simulink model "On_Board_Computer"  (R2024a)
settings: Solver=FixedStepAuto  StartTime=0.0  StopTime=10  FixedStep=sampleTime  RelTol=1e-3
values from neighbouring files (symbols this model uses):
  gains = gainBuilder(kP, kI, kD)    [Data.m]
  params = struct()    [Data.m]
  Q = 0.*eye(12).*1e-0    [Data.m]
  R = diag([(sigma_acc^2).*ones(3,1);      (sigma_gyro^2).*ones(3,1)])    [Data.m]
  sampleTime = 0.01    [Data.m]
libraries: sharedTrackingLibrary x1
settings Model: Creator=matteocolussi  LastModifiedBy=matteocolussi
settings DataIOCC: SaveOutput=off  SaveTime=off
settings DebuggingCC: ParameterPrecisionLossMsg=none
settings ModelReferenceCC: UseModelRefSolver=on

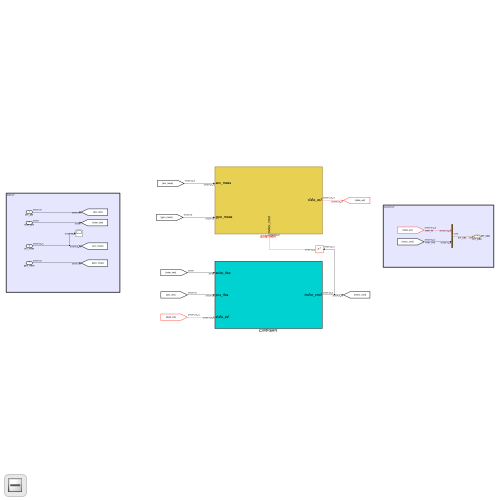
[thumbnail: Simulink's stored preview of the top-level diagram]
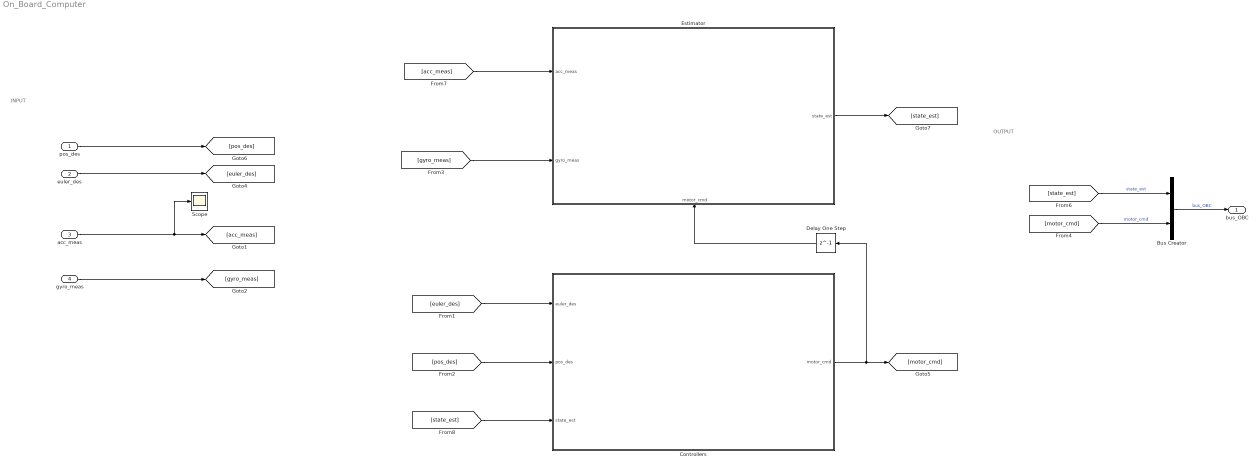
== system On_Board_Computer ==
  note: INPUT
  note: OUTPUT
  pos_des : Inport  OutDataTypeStr=double  PortDimensions=3
  euler_des : Inport  Port=2  OutDataTypeStr=double  PortDimensions=1
  acc_meas : Inport  Port=3  OutDataTypeStr=double  PortDimensions=[3 1]  SampleTime=0
  gyro_meas : Inport  Port=4  OutDataTypeStr=double  PortDimensions=3  SampleTime=0
  Bus Creator : BusCreator  Inputs=2  OutDataTypeStr=Bus: bus_OBC
  Controllers : Subsystem
  Delay One Step : Delay  DelayLength=1
  Estimator : Subsystem
      settings: PortSchema="{\"entries\":[{\"content\":{\"sides\":[{\"content\":{\"connectorIds\":[\"In1\",\"In2\"]},\"type\":\"ConnectorPlacement.EquallySpacedRectSide\",\"uuid\":\"d977f4b7-c562-4aca-a182-8854d6f84319\"},{\"content\":{\"connectorIds\":[\"Out1\"],\"side\":\"RIGHT\"},\"type\":\"ConnectorPlacement.EquallySpacedRectSide\",\"uuid\":\"5ec2f9b4-7086-4916-9bca-a6bf4e760209\"},{\"content\":{\"side\":\"TOP\"},\"type\":\"ConnectorPlacement.EquallySpacedRectSide\",\"uuid\":\"f97c9147-b60d-497a-8876-5f5880fb5fe3\"},{\"content\":{\"connectorIds\":[\"In3\"],\"side\":\"BOTTOM\"},\"type\":\"ConnectorPlacement.EquallySpacedRectSide\",\"uuid\":\"4e01cfcf-7d04-45a0-a360-97a990265c59\"}]},\"type\":\"ConnectorPlacement.EquallySpacedConnector\",\"uuid\":\"f1c31a70-7567-4742-915b-d219842d21d0\"}],\"packageUris\":[\"http://schema.mathworks.com/mf0/Connector/R2020b\"],\"version\":\"1.0\"}"
  Scope : Scope
  bus_OBC : Outport  SignalName=bus_OBC  OutDataTypeStr=Bus: bus_OBC
  wires:
  [euler_des] -> Controllers/1(euler_des)
  [gyro_meas] -> Estimator/2(gyro_meas)
  [acc_meas] -> Estimator/1(acc_meas)
  [pos_des] -> Controllers/2(pos_des)
  Estimator/1(state_est) -> [state_est]
  Controllers/1(motor_cmd) -> Delay One Step/1, [motor_cmd]
  Delay One Step/1 -> Estimator/3(motor_cmd)
  [state_est] -> Controllers/3(state_est)
  [state_est] -> Bus Creator/1  "state_est"
  [motor_cmd] -> Bus Creator/2  "motor_cmd"
  Bus Creator/1 -> bus_OBC/1  "bus_OBC"
  pos_des/1 -> [pos_des]
  euler_des/1 -> [euler_des]
  acc_meas/1 -> [acc_meas], Scope/1
  gyro_meas/1 -> [gyro_meas]

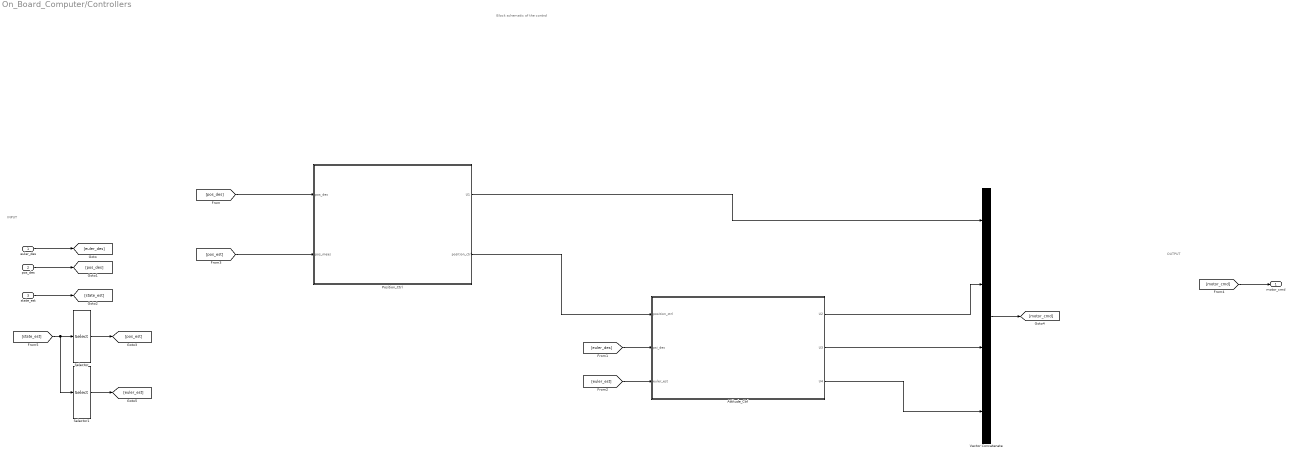
== system On_Board_Computer/Controllers ==
  note: INPUT
  note: OUTPUT
  note: Block schematic of the control
  euler_des : Inport
  pos_des : Inport  Port=2
  state_est : Inport  Port=3
  Attitude_Ctrl : Subsystem
  Position_Ctrl : Subsystem
  Selector : Selector  InputPortWidth=12  IndexOptions=Index vector (dialog)  Indices=1:3  OutputSizes=1
  Selector1 : Selector  InputPortWidth=12  IndexOptions=Index vector (dialog)  Indices=7:9  OutputSizes=1
  Vector Concatenate : Concatenate  NumInputs=4
  motor_cmd : Outport
  wires:
  [euler_des] -> Attitude_Ctrl/2(psi_des)
  Vector Concatenate/1 -> [motor_cmd]
  Attitude_Ctrl/3(U4) -> Vector Concatenate/4
  Attitude_Ctrl/2(U3) -> Vector Concatenate/3
  Attitude_Ctrl/1(U2) -> Vector Concatenate/2
  Position_Ctrl/1(U1) -> Vector Concatenate/1
  Position_Ctrl/2(position_ctrl) -> Attitude_Ctrl/1(position_ctrl)
  [pos_des] -> Position_Ctrl/1(pos_des)
  [pos_est] -> Position_Ctrl/2(pos_meas)
  [motor_cmd] -> motor_cmd/1
  [euler_est] -> Attitude_Ctrl/3(euler_est)
  state_est/1 -> [state_est]
  Selector/1 -> [pos_est]
  pos_des/1 -> [pos_des]
  euler_des/1 -> [euler_des]
  [state_est] -> Selector1/1, Selector/1
  Selector1/1 -> [euler_est]

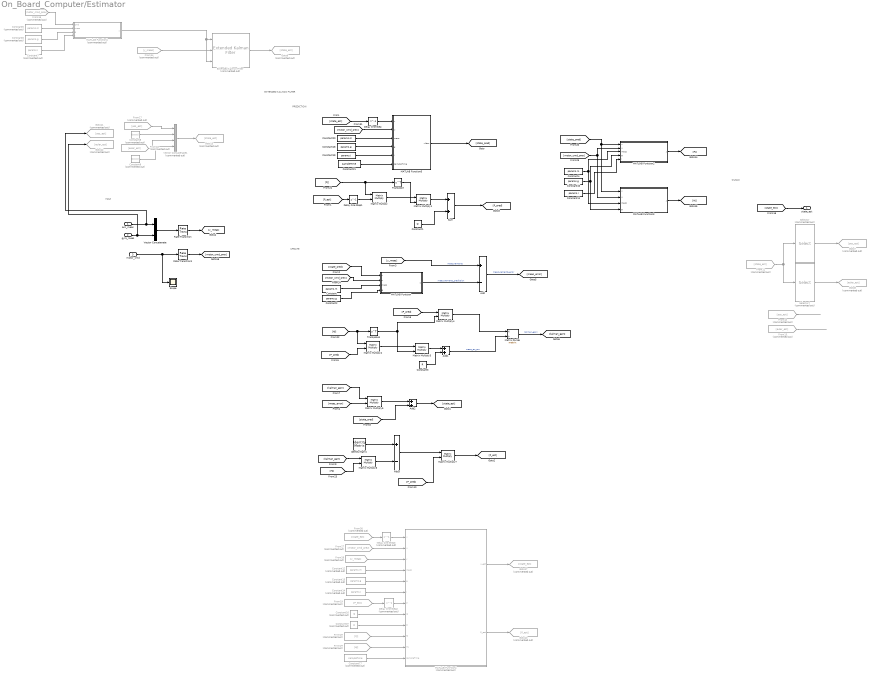
== system On_Board_Computer/Estimator ==
  note: Output
  note: Input
  note: UPDATE
  note: PREDICTION
  note: EXTENDED KALMAN FILTER
  acc_meas : Inport
  gyro_meas : Inport  Port=2
  motor_cmd : Inport  Port=3
  Add : Sum  Inputs=+-
  Add1 : Sum
  Add2 : Sum
  Add3 : Sum  Inputs=+-
  Constant : Constant  Value=params.m
  Constant1 : Constant  Value=Q
  Constant10 : Constant  Value=params.g
  Constant11 : Constant  Value=params.I
  Constant12 : Constant  Commented=on  Value=params.m
  Constant13 : Constant  Commented=on  Value=params.g
  Constant14 : Constant  Commented=on  Value=params.I
  Constant15 : Constant  Commented=on  Value=R
  Constant16 : Constant  Commented=on  Value=Q
  Constant17 : Constant  Commented=on  Value=sampleTime
  Constant18 : Constant  Value=params.g
  Constant19 : Constant  Value=params.I
  Constant2 : Constant  Value=params.g
  Constant20 : Constant  Value=params.m
  Constant21 : Constant  Value=sampleTime
  Constant3 : Constant  Value=R
  Constant4 : Constant  Value=params.m
  Constant5 : Constant  Commented=on  Value=params.m
  Constant6 : Constant  Commented=on  Value=params.g
  Constant7 : Constant  Commented=on  Value=params.I
  Constant8 : Constant  Commented=on  Value=[0;0;0]
  Constant9 : Constant  Commented=on  Value=[0;0;0]
  Delay One Step : Delay  DelayLength=1
  Delay One Step1 : Delay  DelayLength=1
  Delay One Step2 : Delay  Commented=on  DelayLength=1
  Delay One Step3 : Delay  Commented=on  DelayLength=1
  Extended Kalman Filter : sharedTrackingLibrary/Extended Kalman Filter  Commented=on  StateTransitionFcn=stateFunction  HasStateTransitionJacobianFcn=off  HasAdditiveProcessNoise=Additive  ProcessNoise=Q  HasTimeVaryingProcessNoise=off  HasStateTransitionFcnExtraArgument=1  InitialState=zeros(12,1)  InitialStateCovariance=P_est  MeasurementFcn1=measFunction  HasMeasurementJacobianFcn1=off  HasMeasurementEnablePort1=off  HasAdditiveMeasurementNoise1=Additive  MeasurementNoise1=R  HasTimeVaryingMeasurementNoise1=off  HasMeasurementFcnExtraArgument1=1  HasMeasurementWrapping1=off  MeasurementFcn2=myMeasurementFcn  HasMeasurementJacobianFcn2=off  HasMeasurementEnablePort2=off  HasAdditiveMeasurementNoise2=Additive  MeasurementNoise2=1  HasTimeVaryingMeasurementNoise2=off  HasMeasurementFcnExtraArgument2=0  HasMeasurementWrapping2=off  MeasurementFcn3=myMeasurementFcn  HasMeasurementJacobianFcn3=off  HasMeasurementEnablePort3=off  HasAdditiveMeasurementNoise3=Additive  MeasurementNoise3=1  HasTimeVaryingMeasurementNoise3=off  HasMeasurementFcnExtraArgument3=0  HasMeasurementWrapping3=off  MeasurementFcn4=myMeasurementFcn  HasMeasurementJacobianFcn4=off  HasMeasurementEnablePort4=off  HasAdditiveMeasurementNoise4=Additive  MeasurementNoise4=1  HasTimeVaryingMeasurementNoise4=off  HasMeasurementFcnExtraArgument4=0  HasMeasurementWrapping4=off  MeasurementFcn5=myMeasurementFcn  HasMeasurementJacobianFcn5=off  HasMeasurementEnablePort5=off  HasAdditiveMeasurementNoise5=Additive  MeasurementNoise5=1  HasTimeVaryingMeasurementNoise5=off  HasMeasurementFcnExtraArgument5=0  HasMeasurementWrapping5=off  EnableMultirate=off  StateTransitionFcnSampleTime=1  MeasurementFcn1SampleTime=1  MeasurementFcn2SampleTime=1  MeasurementFcn3SampleTime=1  MeasurementFcn4SampleTime=1  MeasurementFcn5SampleTime=1  UseCurrentEstimator=on  OutputStateCovariance=off  DataType=double  SampleTime=sampleTime  NumberOfMeasurements=1
  From11 : From  Commented=on  GotoTag=state_est
  From12 : From  Commented=on  GotoTag=pos_est
  From13 : From  Commented=on  GotoTag=euler_est
  From14 : From  Commented=on  GotoTag=y_meas
  From15 : From  Commented=on  GotoTag=motor_cmd_prev
  From17 : From  Commented=on  GotoTag=pos_est
  From18 : From  Commented=on  GotoTag=euler_est
  From19 : From  Commented=on  GotoTag=P_est
  From26 : From  Commented=on  GotoTag=y_meas
  From27 : From  Commented=on  GotoTag=motor_cmd_prev
  From28 : From  Commented=on  GotoTag=FJ
  From29 : From  Commented=on  GotoTag=HJ
  From30 : From  Commented=on  GotoTag=state_est
  Goto10 : Goto  Commented=on  GotoTag=P_est
  Goto11 : Goto  Commented=on  GotoTag=pos_est
  Goto12 : Goto  Commented=on  GotoTag=euler_est
  Goto13 : Goto  Commented=on  GotoTag=state_est
  Goto17 : Goto  Commented=on  GotoTag=state_est
  Goto7 : Goto  Commented=on  GotoTag=pos_est
  Goto8 : Goto  Commented=on  GotoTag=euler_est
  Goto9 : Goto  Commented=on  GotoTag=state_est
  IdentityMatrix : IdentityMatrix  OutputDimensions=[12,12]  SampleTime=inf
  MATLAB Function : MATLAB Function  TreatAsAtomicUnit=on
  MATLAB Function1 : MATLAB Function  Commented=on  TreatAsAtomicUnit=on
  MATLAB Function2 : MATLAB Function  TreatAsAtomicUnit=on
  MATLAB Function3 : MATLAB Function  TreatAsAtomicUnit=on
  MATLAB Function4 : MATLAB Function  Commented=on  TreatAsAtomicUnit=on
  MATLAB Function5 : MATLAB Function  TreatAsAtomicUnit=on
  Matrix Divide : Product  Inputs=*/  Multiplication=Matrix(*)
  Matrix Multiply{,1..7} (8 alike) : Product  Multiplication=Matrix(*)
  Rate Transition : RateTransition  OutPortSampleTime=sampleTime
  Rate Transition1 : RateTransition  OutPortSampleTime=sampleTime
  Scope : Scope
  Selector : Selector  Commented=on  InputPortWidth=12  IndexOptions=Index vector (dialog)  Indices=1:3  OutputSizes=1
  Selector1 : Selector  Commented=on  InputPortWidth=12  IndexOptions=Index vector (dialog)  Indices=7:9  OutputSizes=1
  Sum : Sum
  Transpose : Math  Operator=transpose
  Transpose1 : Math  Operator=transpose
  Vector Concatenate : Concatenate
  Vector Concatenate1 : Concatenate  Commented=on  NumInputs=4
  state_est : Outport
  wires:
  acc_meas/1 -> Vector Concatenate/1, Goto11/1
  gyro_meas/1 -> Vector Concatenate/2, Goto12/1
  [state_est] -> Delay One Step/1
  Delay One Step/1 -> MATLAB Function5/1(x)
  [P_est] -> Delay One Step1/1
  Delay One Step1/1 -> Matrix Multiply/2
  Matrix Multiply/1 -> Matrix Multiply1/1
  [FJ] -> Transpose/1, Matrix Multiply/1
  Transpose/1 -> Matrix Multiply1/2
  Matrix Multiply1/1 -> Sum/1
  Constant1/1 -> Sum/2
  Sum/1 -> [P_pred]
  [state_pred] -> MATLAB Function/1(x)
  MATLAB Function/1(z) -> Add/2  "measurements_prediction"
  Vector Concatenate/1 -> Rate Transition/1
  [y_meas] -> Add/1  "measurements"
  Add/1 -> [meas_error]  "measurements_error"
  [P_pred] -> Matrix Multiply2/2
  [HJ] -> Matrix Multiply2/1, Transpose1/1
  Matrix Multiply2/1 -> Matrix Multiply3/1
  Transpose1/1 -> Matrix Multiply4/2, Matrix Multiply3/2
  Matrix Multiply3/1 -> Add1/1
  Constant3/1 -> Add1/2
  Add1/1 -> Matrix Divide/2  "meas_err_cov"
  [P_pred] -> Matrix Multiply4/1
  Matrix Multiply4/1 -> Matrix Divide/1
  Matrix Divide/1 -> [kalman_gain]  "kalman_gain"
  [meas_error] -> Matrix Multiply5/2
  [kalman_gain] -> Matrix Multiply5/1
  Matrix Multiply5/1 -> Add2/1
  [state_pred] -> Add2/2
  Add2/1 -> [state_est]
  IdentityMatrix/1 -> Add3/1
  [kalman_gain] -> Matrix Multiply6/1
  [HJ] -> Matrix Multiply6/2
  Matrix Multiply6/1 -> Add3/2
  Add3/1 -> Matrix Multiply7/1
  Matrix Multiply7/1 -> [P_est]
  [P_pred] -> Matrix Multiply7/2
  From11/1 -> Selector1/1, Selector/1
  Selector/1 -> Goto7/1
  Selector1/1 -> Goto8/1
  From12/1 -> ?
  From13/1 -> ?
  Extended Kalman Filter/1 -> Goto9/1
  motor_cmd/1 -> Scope/1, Rate Transition1/1
  From14/1 -> Extended Kalman Filter/2
  Rate Transition/1 -> [y_meas]
  Rate Transition1/1 -> [motor_cmd_prev]
  From15/1 -> MATLAB Function1/1(cmd)
  Constant5/1 -> MATLAB Function1/2(mass)
  Constant6/1 -> MATLAB Function1/3(g)
  Constant7/1 -> MATLAB Function1/4(I)
  MATLAB Function1/1(y) -> Extended Kalman Filter/3, Extended Kalman Filter/1
  [state_est] -> state_est/1
  From17/1 -> Vector Concatenate1/1
  Constant8/1 -> Vector Concatenate1/2
  From18/1 -> Vector Concatenate1/3
  Constant9/1 -> Vector Concatenate1/4
  Vector Concatenate1/1 -> Goto13/1
  [motor_cmd_prev] -> MATLAB Function3/2(u), MATLAB Function2/2(u)
  [state_pred] -> MATLAB Function3/1(x), MATLAB Function2/1(x)
  MATLAB Function2/1(J) -> [FJ]
  MATLAB Function3/1(J) -> [HJ]
  [motor_cmd_prev] -> MATLAB Function/2(u)
  Constant/1 -> MATLAB Function/3(mass)
  Constant2/1 -> MATLAB Function/4(g)
  Constant4/1 -> MATLAB Function3/3(mass), MATLAB Function2/3(mass)
  Constant10/1 -> MATLAB Function3/4(g), MATLAB Function2/4(g)
  Constant11/1 -> MATLAB Function2/5(I)
  MATLAB Function4/2(P_est) -> Goto10/1
  MATLAB Function4/1(x_est) -> Goto17/1
  From19/1 -> Delay One Step2/1
  Delay One Step2/1 -> MATLAB Function4/7(P)
  Constant13/1 -> MATLAB Function4/5(g)
  Constant12/1 -> MATLAB Function4/4(mass)
  Constant14/1 -> MATLAB Function4/6(I)
  From26/1 -> MATLAB Function4/3(y)
  From27/1 -> MATLAB Function4/2(u)
  Constant15/1 -> MATLAB Function4/9(R)
  Constant16/1 -> MATLAB Function4/8(Q)
  From28/1 -> MATLAB Function4/10(FJ)
  From29/1 -> MATLAB Function4/11(HJ)
  From30/1 -> Delay One Step3/1
  Delay One Step3/1 -> MATLAB Function4/1(x)
  Constant17/1 -> MATLAB Function4/12(sampleTime)
  MATLAB Function5/1(xNew) -> [state_pred]
  [motor_cmd_prev] -> MATLAB Function5/2(u)
  Constant20/1 -> MATLAB Function5/3(mass)
  Constant18/1 -> MATLAB Function5/4(g)
  Constant19/1 -> MATLAB Function5/5(I)
  Constant21/1 -> MATLAB Function5/6(sampleTime)

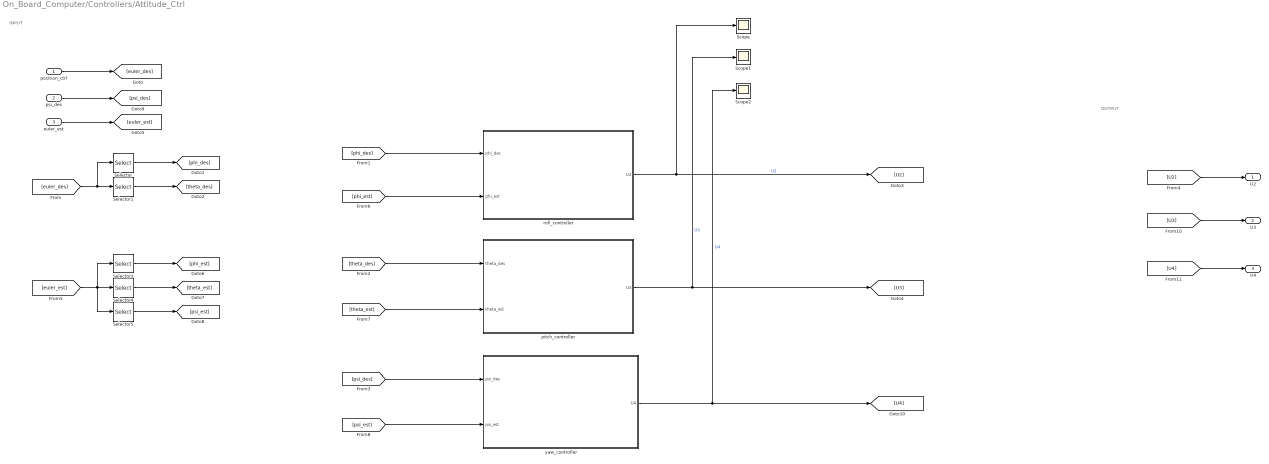
== system On_Board_Computer/Controllers/Attitude_Ctrl ==
  note: INPUT
  note: OUTPUT
  position_ctrl : Inport
  psi_des : Inport  Port=2
  euler_est : Inport  Port=3
  Scope : Scope
  Scope1 : Scope
  Scope2 : Scope
  Selector : Selector  InputPortWidth=2  IndexOptions=Index vector (dialog)  Indices=1  OutputSizes=1
  Selector1 : Selector  InputPortWidth=2  IndexOptions=Index vector (dialog)  Indices=2  OutputSizes=1
  Selector3 : Selector  InputPortWidth=3  IndexOptions=Index vector (dialog)  Indices=1  OutputSizes=1
  Selector4 : Selector  InputPortWidth=3  IndexOptions=Index vector (dialog)  Indices=2  OutputSizes=1
  Selector5 : Selector  InputPortWidth=3  IndexOptions=Index vector (dialog)  Indices=3  OutputSizes=1
  pitch_controller : Subsystem
  roll_controller : Subsystem
  yaw_controller : Subsystem
  U2 : Outport
  U3 : Outport  Port=2
  U4 : Outport  Port=3
  wires:
  psi_des/1 -> [psi_des]
  [U4] -> U4/1
  [U3] -> U3/1
  [U2] -> U2/1
  Selector3/1 -> [phi_est]
  Selector5/1 -> [psi_est]
  Selector4/1 -> [theta_est]
  [euler_est] -> Selector3/1, Selector4/1, Selector5/1
  Selector1/1 -> [theta_des]
  [euler_des] -> Selector/1, Selector1/1
  Selector/1 -> [phi_des]
  [psi_est] -> yaw_controller/2(psi_est)
  [theta_est] -> pitch_controller/2(theta_est)
  [phi_est] -> roll_controller/2(phi_est)
  euler_est/1 -> [euler_est]
  yaw_controller/1(U4) -> Scope2/1, [U4]  "U4"
  pitch_controller/1(U3) -> Scope1/1, [U3]  "U3"
  roll_controller/1(U2) -> Scope/1, [U2]  "U2"
  [psi_des] -> yaw_controller/1(psi_des)
  [theta_des] -> pitch_controller/1(theta_des)
  [phi_des] -> roll_controller/1(phi_des)
  position_ctrl/1 -> [euler_des]

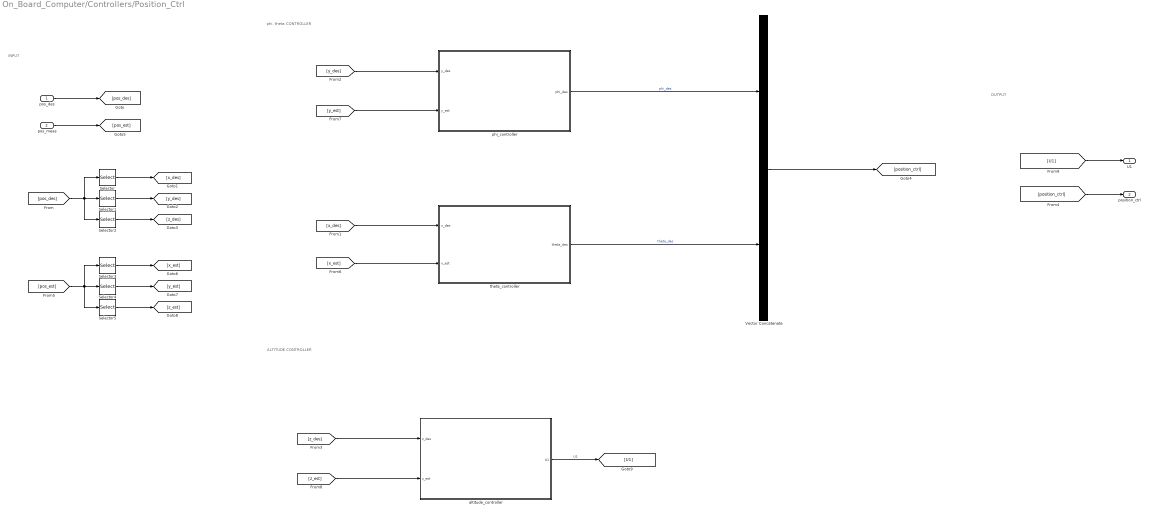
== system On_Board_Computer/Controllers/Position_Ctrl ==
  note: OUTPUT
  note: INPUT
  note: phi, theta CONTROLLER
  note: ALTITUDE CONTROLLER
  pos_des : Inport
  pos_meas : Inport  Port=2
  Selector : Selector  InputPortWidth=3  IndexOptions=Index vector (dialog)  Indices=1  OutputSizes=1
  Selector1 : Selector  InputPortWidth=3  IndexOptions=Index vector (dialog)  Indices=2  OutputSizes=1
  Selector2 : Selector  InputPortWidth=3  IndexOptions=Index vector (dialog)  Indices=3  OutputSizes=1
  Selector3 : Selector  InputPortWidth=3  IndexOptions=Index vector (dialog)  Indices=1  OutputSizes=1
  Selector4 : Selector  InputPortWidth=3  IndexOptions=Index vector (dialog)  Indices=2  OutputSizes=1
  Selector5 : Selector  InputPortWidth=3  IndexOptions=Index vector (dialog)  Indices=3  OutputSizes=1
  Vector Concatenate : Concatenate
  altitude_controller : Subsystem
  phi_controller : Subsystem
  theta_controller : Subsystem
  U1 : Outport
  position_ctrl : Outport  Port=2
  wires:
  phi_controller/1(phi_des) -> Vector Concatenate/1  "phi_des"
  [U1] -> U1/1
  altitude_controller/1(U1) -> [U1]  "U1"
  [z_des] -> altitude_controller/1(z_des)
  [z_est] -> altitude_controller/2(z_est)
  theta_controller/1(theta_des) -> Vector Concatenate/2  "theta_des"
  Vector Concatenate/1 -> [position_ctrl]
  [position_ctrl] -> position_ctrl/1
  [x_est] -> theta_controller/2(x_est)
  [y_des] -> phi_controller/1(y_des)
  [x_des] -> theta_controller/1(x_des)
  [y_est] -> phi_controller/2(y_est)
  Selector2/1 -> [z_des]
  Selector1/1 -> [y_des]
  pos_des/1 -> [pos_des]
  Selector/1 -> [x_des]
  [pos_des] -> Selector/1, Selector1/1, Selector2/1
  Selector5/1 -> [z_est]
  pos_meas/1 -> [pos_est]
  [pos_est] -> Selector3/1, Selector4/1, Selector5/1
  Selector4/1 -> [y_est]
  Selector3/1 -> [x_est]

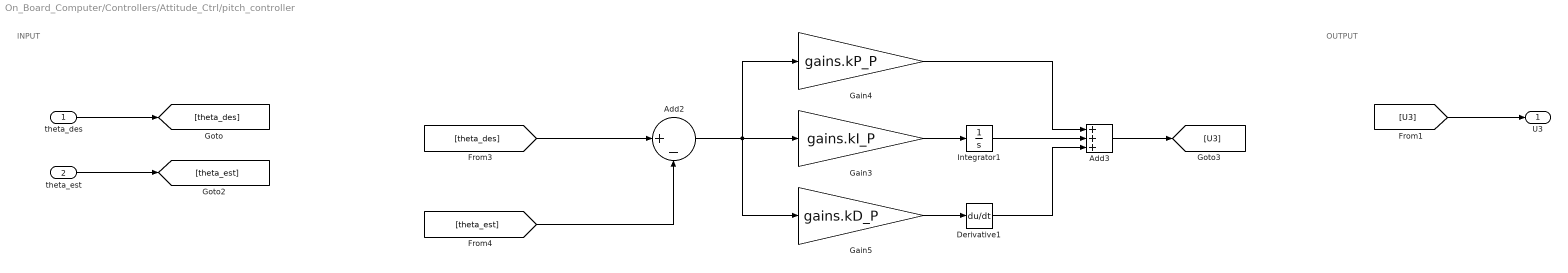
== system On_Board_Computer/Controllers/Attitude_Ctrl/pitch_controller ==
  note: INPUT
  note: OUTPUT
  theta_des : Inport
  theta_est : Inport  Port=2
  Add2 : Sum  Inputs=|+-
  Add3 : Sum  Inputs=+++
  Derivative1 : Derivative
  Gain3 : Gain  Gain=gains.kI_P
  Gain4 : Gain  Gain=gains.kP_P
  Gain5 : Gain  Gain=gains.kD_P
  Integrator1 : Integrator
  U3 : Outport
  wires:
  Gain3/1 -> Integrator1/1
  Gain5/1 -> Derivative1/1
  Add2/1 -> Gain3/1, Gain4/1, Gain5/1
  Integrator1/1 -> Add3/2
  [theta_est] -> Add2/2
  Derivative1/1 -> Add3/3
  Add3/1 -> [U3]
  Gain4/1 -> Add3/1
  [theta_des] -> Add2/1
  theta_est/1 -> [theta_est]
  theta_des/1 -> [theta_des]
  [U3] -> U3/1

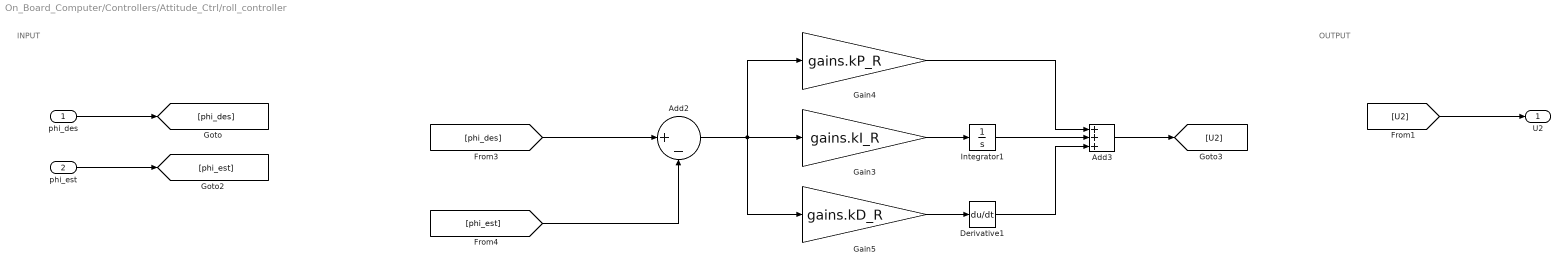
== system On_Board_Computer/Controllers/Attitude_Ctrl/roll_controller ==
  note: INPUT
  note: OUTPUT
  phi_des : Inport
  phi_est : Inport  Port=2
  Add2 : Sum  Inputs=|+-
  Add3 : Sum  Inputs=+++
  Derivative1 : Derivative
  Gain3 : Gain  Gain=gains.kI_R
  Gain4 : Gain  Gain=gains.kP_R
  Gain5 : Gain  Gain=gains.kD_R
  Integrator1 : Integrator
  U2 : Outport
  wires:
  Gain3/1 -> Integrator1/1
  Gain5/1 -> Derivative1/1
  Add2/1 -> Gain3/1, Gain4/1, Gain5/1
  Integrator1/1 -> Add3/2
  [phi_est] -> Add2/2
  Derivative1/1 -> Add3/3
  Add3/1 -> [U2]
  Gain4/1 -> Add3/1
  [phi_des] -> Add2/1
  phi_est/1 -> [phi_est]
  [U2] -> U2/1
  phi_des/1 -> [phi_des]

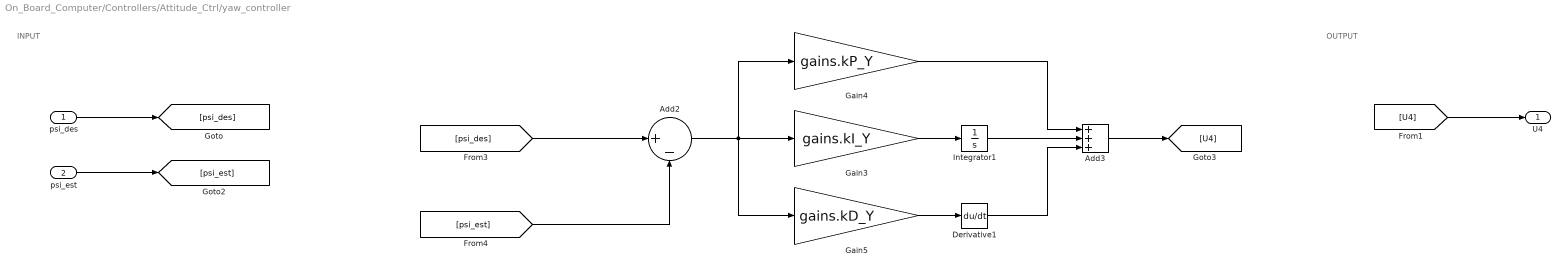
== system On_Board_Computer/Controllers/Attitude_Ctrl/yaw_controller ==
  note: INPUT
  note: OUTPUT
  psi_des : Inport
  psi_est : Inport  Port=2
  Add2 : Sum  Inputs=|+-
  Add3 : Sum  Inputs=+++
  Derivative1 : Derivative
  Gain3 : Gain  Gain=gains.kI_Y
  Gain4 : Gain  Gain=gains.kP_Y
  Gain5 : Gain  Gain=gains.kD_Y
  Integrator1 : Integrator
  U4 : Outport
  wires:
  Gain3/1 -> Integrator1/1
  Gain5/1 -> Derivative1/1
  Add2/1 -> Gain3/1, Gain4/1, Gain5/1
  Integrator1/1 -> Add3/2
  [psi_est] -> Add2/2
  Derivative1/1 -> Add3/3
  Add3/1 -> [U4]
  Gain4/1 -> Add3/1
  [psi_des] -> Add2/1
  psi_est/1 -> [psi_est]
  psi_des/1 -> [psi_des]
  [U4] -> U4/1

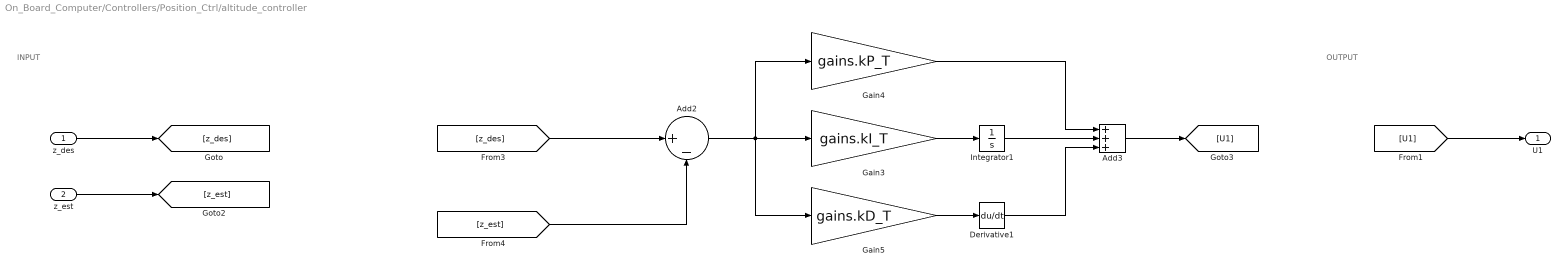
== system On_Board_Computer/Controllers/Position_Ctrl/altitude_controller ==
  note: INPUT
  note: OUTPUT
  z_des : Inport
  z_est : Inport  Port=2
  Add2 : Sum  Inputs=|+-
  Add3 : Sum  Inputs=+++
  Derivative1 : Derivative
  Gain3 : Gain  Gain=gains.kI_T
  Gain4 : Gain  Gain=gains.kP_T
  Gain5 : Gain  Gain=gains.kD_T
  Integrator1 : Integrator
  U1 : Outport
  wires:
  Gain3/1 -> Integrator1/1
  Gain5/1 -> Derivative1/1
  Add2/1 -> Gain3/1, Gain4/1, Gain5/1
  Integrator1/1 -> Add3/2
  [z_est] -> Add2/2
  Derivative1/1 -> Add3/3
  Add3/1 -> [U1]
  Gain4/1 -> Add3/1
  [z_des] -> Add2/1
  z_est/1 -> [z_est]
  z_des/1 -> [z_des]
  [U1] -> U1/1

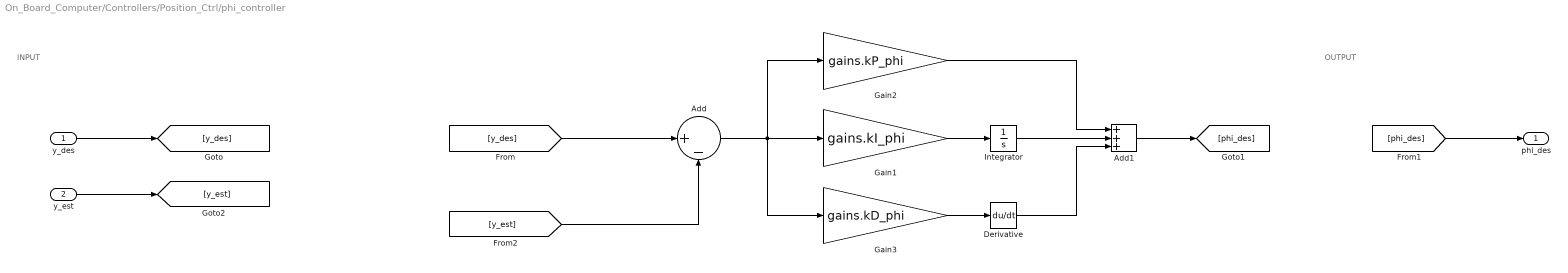
== system On_Board_Computer/Controllers/Position_Ctrl/phi_controller ==
  note: INPUT
  note: OUTPUT
  y_des : Inport
  y_est : Inport  Port=2
  Add : Sum  Inputs=|+-
  Add1 : Sum  Inputs=+++
  Derivative : Derivative
  Gain1 : Gain  Gain=gains.kI_phi
  Gain2 : Gain  Gain=gains.kP_phi
  Gain3 : Gain  Gain=gains.kD_phi
  Integrator : Integrator
  phi_des : Outport
  wires:
  Gain3/1 -> Derivative/1
  Add1/1 -> [phi_des]
  Derivative/1 -> Add1/3
  Gain2/1 -> Add1/1
  Add/1 -> Gain1/1, Gain2/1, Gain3/1
  Gain1/1 -> Integrator/1
  Integrator/1 -> Add1/2
  [y_est] -> Add/2
  y_est/1 -> [y_est]
  y_des/1 -> [y_des]
  [y_des] -> Add/1
  [phi_des] -> phi_des/1

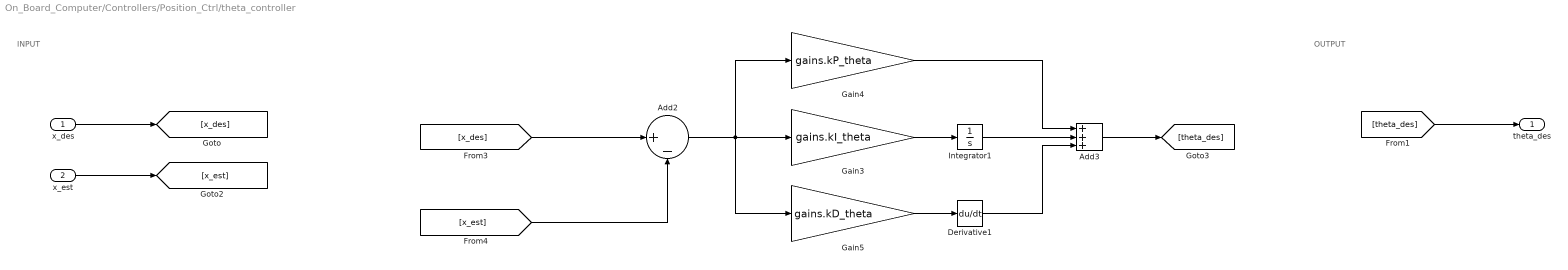
== system On_Board_Computer/Controllers/Position_Ctrl/theta_controller ==
  note: INPUT
  note: OUTPUT
  x_des : Inport
  x_est : Inport  Port=2
  Add2 : Sum  Inputs=|+-
  Add3 : Sum  Inputs=+++
  Derivative1 : Derivative
  Gain3 : Gain  Gain=gains.kI_theta
  Gain4 : Gain  Gain=gains.kP_theta
  Gain5 : Gain  Gain=gains.kD_theta
  Integrator1 : Integrator
  theta_des : Outport
  wires:
  Gain3/1 -> Integrator1/1
  Gain5/1 -> Derivative1/1
  Add2/1 -> Gain3/1, Gain4/1, Gain5/1
  Integrator1/1 -> Add3/2
  [x_est] -> Add2/2
  Derivative1/1 -> Add3/3
  Add3/1 -> [theta_des]
  Gain4/1 -> Add3/1
  [x_des] -> Add2/1
  x_est/1 -> [x_est]
  [theta_des] -> theta_des/1
  x_des/1 -> [x_des]

== matlab function On_Board_Computer/Estimator/MATLAB Function1 ==
  data: cmd input; y output; mass input; g input; I input
function y = manageKalmanFilterInputs(cmd, mass, g, I)

y = zeros(9, 3);
y(1:4, 1) = cmd;
y(5, 1) = mass;
y(6, 1) = g;
y(7:9, 1:3) = I;

== matlab function On_Board_Computer/Estimator/MATLAB Function ==
  data: x input; z output; u input; mass input; g input
function z = h(x, u, mass, g)

% x: x_pred

R_psi = @(x) [cos(x(9)),    -sin(x(9)),     0;
    sin(x(9)),     cos(x(9)),     0;
    0,             0,     1];

R_theta = @(x) [cos(x(8)),      0,      sin(x(8));
    0,      1,              0;
    -sin(x(8)),     0,       cos(x(8))];

R_phi = @(x) [1,        0,              0;
    0,        cos(x(7)),      -sin(x(7));
    0,        sin(x(7)),      cos(x(7))];

rotMat = @(x) R_psi(x) * R_theta(x) * R_phi(x);

% acc = @(x, u) (1/mass).*rotMat(x)*[0; 0; u(1)] + [0; 0; -g];

h = @(x, u) [
    (1/mass).*[0; 0; u(1)] + rotMat(x)'*[0;0;-g];
    x(10:12);
    ];

z = h(x, u);
end

== matlab function On_Board_Computer/Estimator/MATLAB Function2 ==
  data: J output; x input; u input; mass input; g input; I input
function J = JacobianF(x, u, mass, g, I)

R_psi = @(x) [cos(x(9)),    -sin(x(9)),     0;
    sin(x(9)),     cos(x(9)),     0;
    0,             0,     1];

R_theta = @(x) [cos(x(8)),      0,      sin(x(8));
    0,      1,              0;
    -sin(x(8)),     0,       cos(x(8))];

R_phi = @(x) [1,        0,              0;
    0,        cos(x(7)),      -sin(x(7));
    0,        sin(x(7)),      cos(x(7))];

rotMat = @(x) R_psi(x) * R_theta(x) * R_phi(x);

f = @(x, u) [x(4:6);
            (1/mass).*rotMat(x)*[0; 0; u(1)] + [0; 0; -g];
            x(10:12);
            I \ ([u(2); u(3); u(4)] - cross(x(10:12), I*x(10:12)))
            ];

dX = 1e-3;
J = zeros(12, 12);

for i = 1:12 % Row (derive with respect to the i-th component)
    for k = 1:12  % Column
        xEst1 = x;
        xEst2 = x;
        xEst1(k) = x(k) + dX;
        xEst2(k) = x(k) - dX;

        j1 = f(xEst1, u);
        j2 = f(xEst2, u);

        J(i, k) = (j1(i) - j2(i)) / (2 * dX);
    end
end
end

== matlab function On_Board_Computer/Estimator/MATLAB Function3 ==
  data: J output; x input; u input; mass input; g input
function J = JacobianH(x, u, mass, g)

R_psi = @(x) [cos(x(9)),    -sin(x(9)),     0;
    sin(x(9)),     cos(x(9)),     0;
    0,             0,     1];

R_theta = @(x) [cos(x(8)),      0,      sin(x(8));
    0,      1,              0;
    -sin(x(8)),     0,       cos(x(8))];

R_phi = @(x) [1,        0,              0;
    0,        cos(x(7)),      -sin(x(7));
    0,        sin(x(7)),      cos(x(7))];

rotMat = @(x) R_psi(x) * R_theta(x) * R_phi(x);

%acc = @(x, u) (1/mass).*rotMat(x)*[0; 0; u(1)] + [0; 0; -g];

h = @(x, u) [
    (1/mass).*[0; 0; u(1)] + rotMat(x)'*[0;0;-g];
    x(10:12);
    ];


dX = 1e-3;
J = zeros(6, 12);  % 6 osservazioni, 12 variabili di stato

for i = 1:6 % Row (derive with respect to the i-th observation)
    for k = 1:12  % Column
        xEst1 = x;
        xEst2 = x;
        xEst1(k) = x(k) + dX;
        xEst2(k) = x(k) - dX;

        j1 = h(xEst1, u);
        j2 = h(xEst2, u);

        J(i, k) = (j1(i) - j2(i)) / (2 * dX);
    end
end
end

== matlab function On_Board_Computer/Estimator/MATLAB Function4 ==
  data: x input; u input; y input; x_est output; mass input; g input; I input; P input; Q input; R input; FJ input; HJ input; P_est output; sampleTime input
function [x_est, P_est] = kalmanFilter(x, u, y, mass, g, I, P, Q, R, FJ, HJ, sampleTime)

% Functions
R_psi = @(x) [cos(x(9)),    -sin(x(9)),     0;
    sin(x(9)),     cos(x(9)),     0;
    0,             0,     1];

R_theta = @(x) [cos(x(8)),      0,      sin(x(8));
    0,      1,              0;
    -sin(x(8)),     0,       cos(x(8))];

R_phi = @(x) [1,        0,              0;
    0,        cos(x(7)),      -sin(x(7));
    0,        sin(x(7)),      cos(x(7))];

rotMat = @(x) R_psi(x) * R_theta(x) * R_phi(x);

% acc = @(x, u) (1/mass).*rotMat(x)*[0; 0; u(1)] + [0; 0; -g];

f = @(x, u) [x(4:6);
            (1/mass).*rotMat(x)*[0; 0; u(1)] + [0; 0; -g];
            x(10:12);
            I \ ([u(2); u(3); u(4)] - cross(x(10:12), I*x(10:12)))
            ];

h = @(x, u) [
    (1/mass).*[0; 0; u(1)] + rotMat(x)'*[0;0;-g];
    x(10:12);
    ];

% Prediction
x_pred = x + f(x, u).*sampleTime;
P_pred = FJ * P * FJ' + Q;

% Update
y_pred = h(x_pred, u);

Kg = (P_pred * HJ') \ (HJ * P_pred * HJ' + R);

P_est = (eye(12) - Kg*HJ) * P_pred;
x_est = x_pred + (Kg * (y - y_pred));

end

== matlab function On_Board_Computer/Estimator/MATLAB Function5 ==
  data: x input; u input; xNew output; mass input; g input; I input; sampleTime input
function xNew = func(x, u, mass, g, I, sampleTime)

R_psi = @(x) [cos(x(9)),    -sin(x(9)),     0;
    sin(x(9)),     cos(x(9)),     0;
    0,             0,     1];

R_theta = @(x) [cos(x(8)),      0,      sin(x(8));
    0,      1,              0;
    -sin(x(8)),     0,       cos(x(8))];

R_phi = @(x) [1,        0,              0;
    0,        cos(x(7)),      -sin(x(7));
    0,        sin(x(7)),      cos(x(7))];

rotMat = @(x) R_psi(x) * R_theta(x) * R_phi(x);

f = @(x, u) [x(4:6);
            (1/mass).*rotMat(x)*[0; 0; u(1)] + [0; 0; -g];
            x(10:12);
            I \ ([u(2); u(3); u(4)] - cross(x(10:12), I*x(10:12)))
            ];

xNew = x + f(x, u).*sampleTime;

end
